simulink model "simulation_ex10_PID"  (R2023a)
settings: Solver=VariableStepAuto  StartTime=0.0  StopTime=10.0  RelTol=1e-3
values from neighbouring files (symbols this model uses):
  D = sqrt(D)    [ex03.m]    (also in ex05.m = [0; 0]; ex10.m = 0.1; ex11.m = 0; ex11_2.m = [0 0; 0 1])
  M = 1    [ex10.m]
settings Model: Creator=vigro  LastModifiedBy=vigro

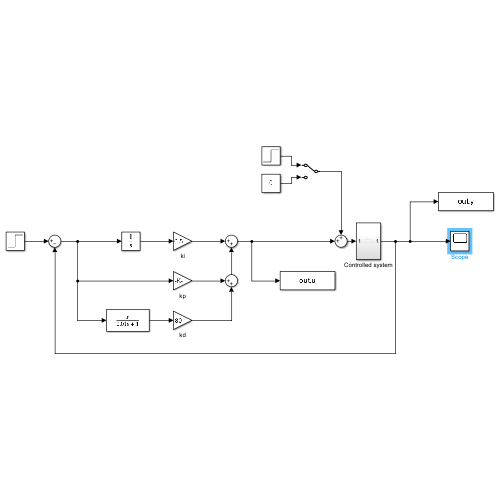
[thumbnail: Simulink's stored preview of the top-level diagram]
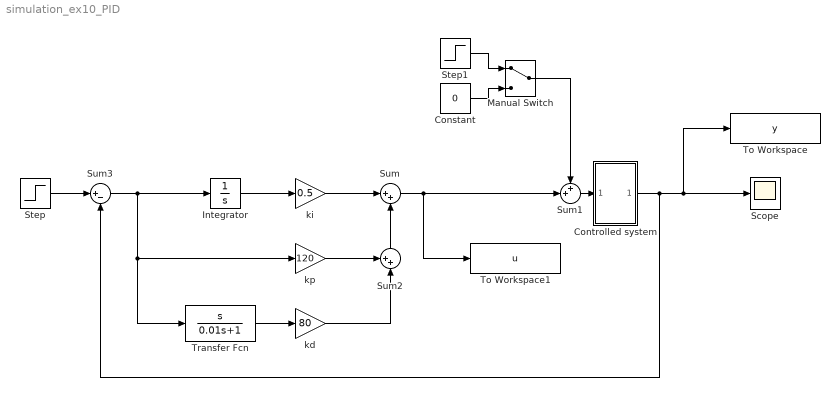
== system simulation_ex10_PID ==
  Constant : Constant  Value=0
  Controlled system : Subsystem
  Integrator : Integrator
  Manual Switch : ManualSwitch
  Scope : Scope
  Step : Step  Time=0  SampleTime=0
  Step1 : Step  SampleTime=0
  Sum : Sum  Inputs=|++
  Sum1 : Sum  Inputs=++|
  Sum2 : Sum  Inputs=++|
  Sum3 : Sum  Inputs=|+-
  To Workspace : ToWorkspace  VariableName=y  SaveFormat=Timeseries  SampleTime=-1
  To Workspace1 : ToWorkspace  VariableName=u  SaveFormat=Timeseries  SampleTime=-1
  Transfer Fcn : TransferFcn  Numerator=[1 0]  Denominator=[0.01 1]
  kd : Gain  Gain=80
  ki : Gain  Gain=0.5
  kp : Gain  Gain=120
  wires:
  kd/1 -> Sum2/2
  Controlled system/1(Out1) -> Scope/1, To Workspace/1, Sum3/2
  Constant/1 -> Manual Switch/2
  Sum3/1 -> kp/1, Transfer Fcn/1, Integrator/1
  Integrator/1 -> ki/1
  Step1/1 -> Manual Switch/1
  kp/1 -> Sum2/1
  Step/1 -> Sum3/1
  Sum/1 -> To Workspace1/1, Sum1/2
  Manual Switch/1 -> Sum1/1
  Transfer Fcn/1 -> kd/1
  Sum1/1 -> Controlled system/1(In1)
  Sum2/1 -> Sum/2
  ki/1 -> Sum/1

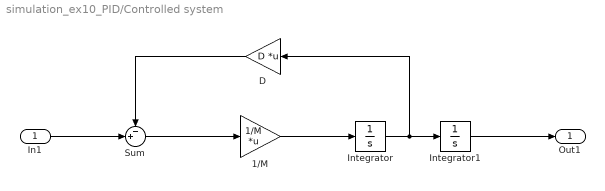
== system simulation_ex10_PID/Controlled system ==
  In1 : Inport
  1/M : Gain  Gain=1/M  Multiplication=Matrix(K*u) (u vector)
  D : Gain  Gain=D  Multiplication=Matrix(K*u) (u vector)
  Integrator : Integrator
  Integrator1 : Integrator
  Sum : Sum  Inputs=-+|
  Out1 : Outport
  wires:
  D/1 -> Sum/1
  Integrator/1 -> D/1, Integrator1/1
  1/M/1 -> Integrator/1
  Sum/1 -> 1/M/1
  In1/1 -> Sum/2
  Integrator1/1 -> Out1/1
